simulink model "E2CdB"  (R2020a)
settings: Solver=ode4  StartTime=0.0  StopTime=10.0  FixedStep=0.001  RelTol=1e-3
settings Model: Creator=megat  LastModifiedBy=megat

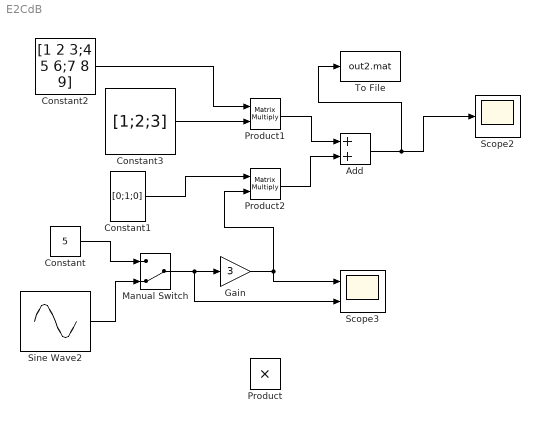
== system E2CdB ==
  Add : Sum
  Constant : Constant  Value=5
  Constant1 : Constant  Value=[0;1;0]  VectorParams1D=off
  Constant2 : Constant  Value=[1 2 3;4 5 6;7 8 9]  VectorParams1D=off
  Constant3 : Constant  Value=[1;2;3]  VectorParams1D=off
  Gain : Gain  Gain=3
  Manual Switch : ManualSwitch  CurrentSetting=0
  Product : Product
  Product1 : Product  Multiplication=Matrix(*)
  Product2 : Product  Multiplication=Matrix(*)
  Scope2 : Scope
  Scope3 : Scope  NumInputPorts=2
  Sine Wave2 : Sin  Amplitude=1.5  Frequency=50  SampleTime=.1
  To File : ToFile  Filename=out2.mat  MatrixName=wwe  SaveFormat=Timeseries
  wires:
  Manual Switch/1 -> Scope3/2, Gain/1
  Gain/1 -> Scope3/1, Product2/2
  Constant/1 -> Manual Switch/1
  Sine Wave2/1 -> Manual Switch/2
  Add/1 -> Scope2/1, To File/1
  Product1/1 -> Add/1
  Product2/1 -> Add/2
  Constant1/1 -> Product2/1
  Constant2/1 -> Product1/1
  Constant3/1 -> Product1/2
